simulink model "MissionProfileGenerator"  (R2023b)
settings: Solver=VariableStepAuto  StartTime=0.0  StopTime=800  RelTol=1e-3
values from neighbouring files (symbols this model uses):
  Dyno_Kt = 0.1041    [ParallelTestBenchParameters.m]
  Dyno_Ratio = 0.44    [ParallelTestBenchParameters.m]
  Power_Map = [0 0 0 0 0 0 0 ... (first row only)    [ParallelTestBenchParameters.m]
  RPM_Governor = [0 1.666666667 3.333333333 5.222227308 6.777784559 8.222223918                 9.111116197 10 10.44444614 10.88889228 12.33334012 13.88888889                 17.00000339 20 23.33333333 26.222229 29.1111162 32.22222222                 36.44444784 40 43.66667853 47.55556742 50.44444614                 53.9999983 58.00000509 60.44444614 64.44445292 68.9999983                 72.66666836 77.00001187 8 ...(+78 chars)    [ParallelTestBenchParameters.m]
  Spd_BP = [0 2000 3000 4000 5000 6000 7500]    [ParallelTestBenchParameters.m]
undefined symbols (not defined in the file or in its folder): rad, s
libraries: SignalEditorBlockLib x4, aerolibconvert2 x2, dspstat3 x1
settings Model: Creator=jwilson  LastModifiedBy=jwilson

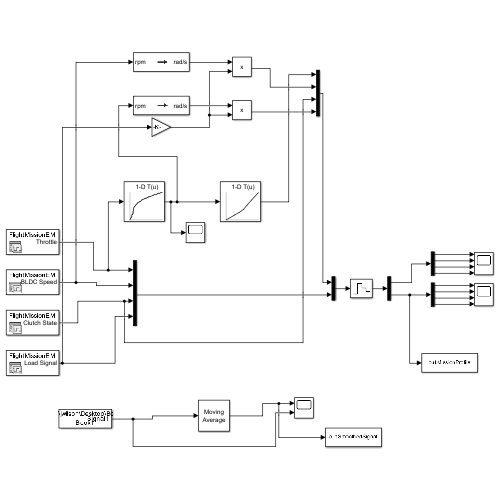
[thumbnail: Simulink's stored preview of the top-level diagram]
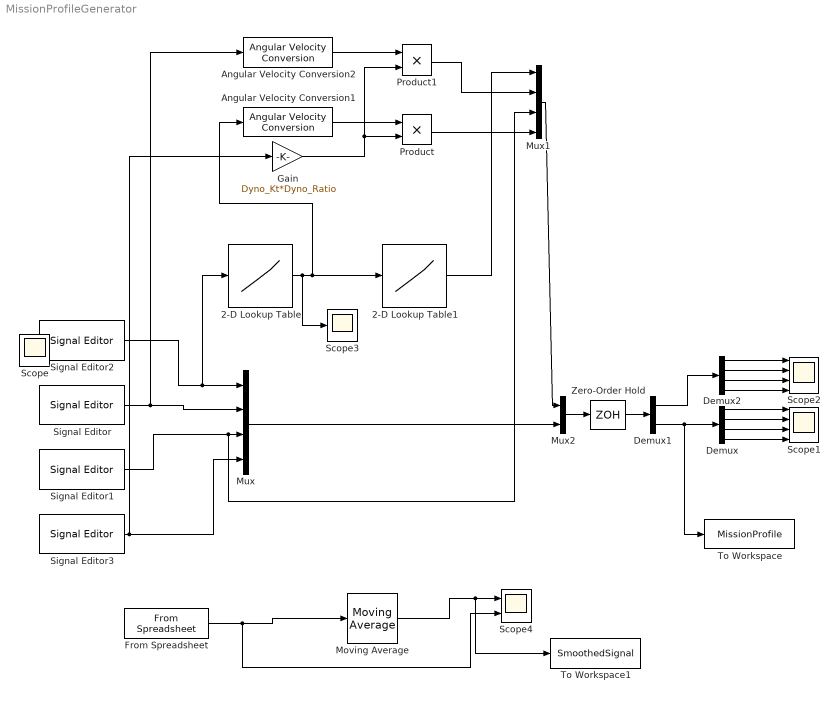
== system MissionProfileGenerator ==
  2-D Lookup Table : Lookup_n-D  NumberOfTableDimensions=1  BreakpointsForDimension1=RPM_Governor(1,:)  BreakpointsForDimension2=[1:3]  Table=RPM_Governor(2,:)  ExtrapMethod=Clip  InternalRulePriority=Speed  RndMeth=Simplest
  2-D Lookup Table1 : Lookup_n-D  NumberOfTableDimensions=1  BreakpointsForDimension1=Spd_BP  BreakpointsForDimension2=[1:3]  Table=Power_Map(12,:)  ExtrapMethod=Clip  InternalRulePriority=Speed  RndMeth=Simplest
  Angular Velocity Conversion1 : aerolibconvert2/Angular Velocity Conversion  IU=rpm  OU=rad/s
  Angular Velocity Conversion2 : aerolibconvert2/Angular Velocity Conversion  IU=rpm  OU=rad/s
  Demux : Demux
  Demux1 : Demux  Outputs=2
  Demux2 : Demux
  From Spreadsheet : FromSpreadsheet  FileName=C:\Users\jwilson\Desktop\Book1.csv  SheetName=Book1
  Gain : Gain  Gain=Dyno_Kt*Dyno_Ratio
  Moving Average : dspstat3/Moving Average  Method=Sliding window  ForgettingFactorPort=off  SpecifyWindowLength=on  WindowLength=4  OverlapLength=3  AllowArbitraryInputLength=off  ForgettingFactor=0.9  SimulateUsing=Code generation
  Mux : Mux
  Mux1 : Mux
  Mux2 : Mux  Inputs=2
  Product : Product
  Product1 : Product
  Scope1 : Scope  NumInputPorts=4
  Scope2 : Scope  NumInputPorts=4
  Scope3 : Scope
  Scope4 : Scope  NumInputPorts=2
  Signal Editor : SignalEditorBlockLib/Signal Editor  FileName=BLDC Speed Signal.mat  ActiveScenario=FlightMissionEM  ActiveSignal=BLDC Speed  IsBus=off  OutputBusObjectStr=Bus: BusObject  SampleTime=0  ZeroCross=off  OutputAfterFinalValue=Setting to zero  Unit=inherit  PreserveSignalName=on  ApplySigPropsToAllScenarios=on  ApplySigPropsToAllSignals=off
  Signal Editor1 : SignalEditorBlockLib/Signal Editor  FileName=Clutch Signal.mat  ActiveScenario=FlightMissionEM  ActiveSignal=Clutch State  IsBus=off  OutputBusObjectStr=Bus: BusObject  SampleTime=0  ZeroCross=off  OutputAfterFinalValue=Setting to zero  Unit=inherit  PreserveSignalName=on  ApplySigPropsToAllScenarios=on  ApplySigPropsToAllSignals=off
  Signal Editor2 : SignalEditorBlockLib/Signal Editor  FileName=Throttle Signal.mat  ActiveScenario=FlightMissionEM  ActiveSignal=Throttle  IsBus=off  OutputBusObjectStr=Bus: BusObject  SampleTime=0  ZeroCross=off  OutputAfterFinalValue=Setting to zero  Unit=inherit  PreserveSignalName=on  ApplySigPropsToAllScenarios=on  ApplySigPropsToAllSignals=off
  Signal Editor3 : SignalEditorBlockLib/Signal Editor  FileName=Load Signal.mat  ActiveScenario=FlightMissionEM  ActiveSignal=Load Signal  IsBus=off  OutputBusObjectStr=Bus: BusObject  SampleTime=0  ZeroCross=off  OutputAfterFinalValue=Setting to zero  Unit=inherit  PreserveSignalName=on  ApplySigPropsToAllScenarios=on  ApplySigPropsToAllSignals=off
  To Workspace : ToWorkspace  VariableName=MissionProfile  SampleTime=-1
  To Workspace1 : ToWorkspace  VariableName=SmoothedSignal  SampleTime=-1
  Zero-Order Hold : ZeroOrderHold  SampleTime=0.1
  Scope : Scope
  wires:
  Demux/1 -> Scope1/1
  Demux/2 -> Scope1/2
  Demux/3 -> Scope1/3
  Demux/4 -> Scope1/4
  Signal Editor2/1 -> 2-D Lookup Table/1, Mux/1
  Signal Editor/1 -> Angular Velocity Conversion2/1, Mux/2
  Signal Editor1/1 -> Mux1/3, Mux/3
  Signal Editor3/1 -> Mux/4, Gain/1
  2-D Lookup Table/1 -> Scope3/1, Angular Velocity Conversion1/1, 2-D Lookup Table1/1
  Angular Velocity Conversion1/1 -> Product/1
  Angular Velocity Conversion2/1 -> Product1/1
  Gain/1 -> Product1/2, Product/2
  2-D Lookup Table1/1 -> Mux1/1
  Product1/1 -> Mux1/2
  Product/1 -> Mux1/4
  Mux2/1 -> Zero-Order Hold/1
  Mux1/1 -> Mux2/1
  Mux/1 -> Mux2/2
  Zero-Order Hold/1 -> Demux1/1
  Demux1/2 -> To Workspace/1, Demux/1
  Demux2/2 -> Scope2/2
  Demux2/3 -> Scope2/3
  Demux2/1 -> Scope2/1
  Demux2/4 -> Scope2/4
  Demux1/1 -> Demux2/1
  From Spreadsheet/1 -> Scope4/2, Moving Average/1
  Moving Average/1 -> To Workspace1/1, Scope4/1
